simulink model "quad_tank_plant"  (R2026a)
settings: Solver=ode4  StopTime=inf
values from neighbouring files (symbols this model uses):
  a1 = (a11 + a12)/2    [areas.m]    (also in parametros.m = 0.0006136)
  A2 = 0.159    [parametros.m]
  a2 = mean([a21 a22],2)    [areas.m]    (also in parametros.m = 0.00054678)
  A3 = 0.159    [parametros.m]
  a3 = mean([a31 a32],2)    [areas.m]    (also in parametros.m = 0.00035752; prbs_calc_L3.m = 0.00035752; ti_calc.m = 0.00035752)
  A4 = 0.159    [parametros.m]
  a4 = mean([a41 a42],2)    [areas.m]    (also in parametros.m = 0.0004182; ti_calc.m = 0.0004182)
  g = 9.81    [areas.m]    (also in parametros.m; prbs_calc_L3.m; ti_calc.m)
  gamma1 = 0.455    [areas.m]    (also in parametros.m)
  gamma2 = 0.4195    [areas.m]    (also in parametros.m)
  h_max = 0.6    [areas.m]    (also in parametros.m)
  k1 = q_max    (= 0.0017)    [areas.m]    (also in parametros.m)
  k2 = q_max    (= 0.0017)    [areas.m]    (also in parametros.m)
  q_max = 0.0017    [areas.m]    (also in parametros.m)
undefined symbols (not defined in the file or in its folder): A1
libraries: opcualib x2
settings Model: Creator=agusc  LastModifiedBy=agusc

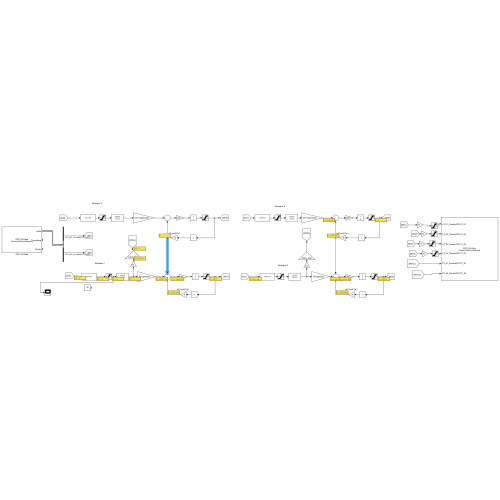
[thumbnail: Simulink's stored preview of the top-level diagram]
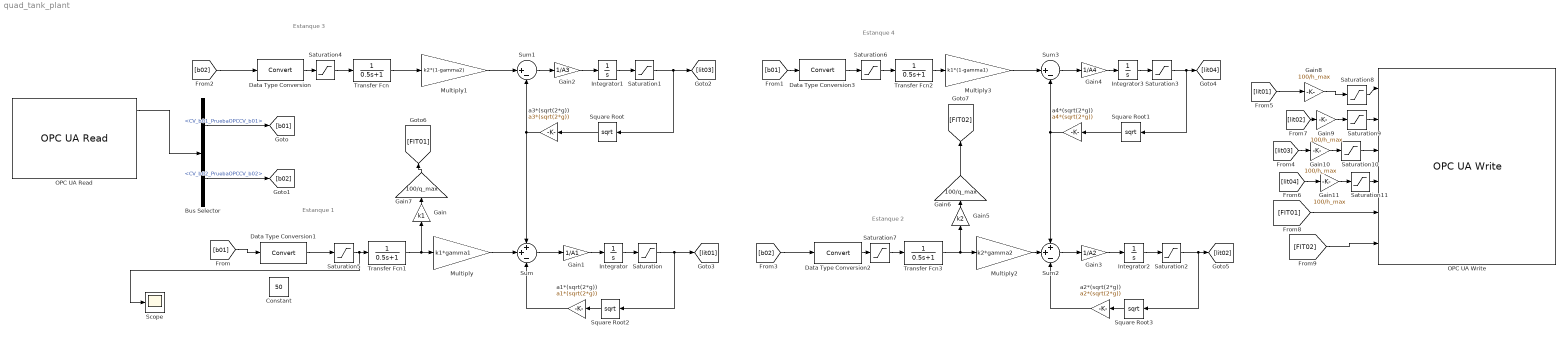
== system quad_tank_plant ==
  note: Estanque 2
  note: Estanque 4
  note: Estanque 3
  note: Estanque 1
  Bus Selector : BusSelector  OutputSignals=CV_b01_PruebaOPCCV_b01,CV_b02_PruebaOPCCV_b02
  Constant : Constant  Value=50
  Data Type Conversion{,1..3} (4 alike) : DataTypeConversion  SaturateOnIntegerOverflow=off  RndMeth=Floor
  Gain : Gain  Gain=k1
  Gain1 : Gain  Gain=1/A1
  Gain{8..11} (4 alike) : Gain  Gain=100/h_max
  Gain2 : Gain  Gain=1/A3
  Gain3 : Gain  Gain=1/A2
  Gain4 : Gain  Gain=1/A4
  Gain5 : Gain  Gain=k2
  Gain6 : Gain  Gain=100/q_max
  Gain7 : Gain  Gain=100/q_max
  Integrator{,1..3} (4 alike) : Integrator
  Multiply : Gain  Gain=k1*gamma1
  Multiply1 : Gain  Gain=k2*(1-gamma2)
  Multiply2 : Gain  Gain=k2*gamma2
  Multiply3 : Gain  Gain=k1*(1-gamma1)
  OPC UA Read : opcualib/OPC UA Read  SelectedServer=FactoryTalkLinxGateway  ServerList=FactoryTalkLinxGateway  NodeList={ '1', 'CV_b01', '2', '[Prueba OPC]CV_b01', 'off'; '2', 'CV_b02', '2', '[Prueba OPC]CV_b02', 'off' }  ShowQualityPort=on  ShowTimestampPort=on  ShowTimestampPortAs=Seconds since start  SampleTime=-1
  OPC UA Write : opcualib/OPC UA Write  SelectedServer=FactoryTalkLinxGateway  ServerList=FactoryTalkLinxGateway  SampleTime=-1  NodeList={ '1', 'LIT_01', '2', '[Prueba OPC]LIT_01', 'off'; '2', 'LIT_02', '2', '[Prueba OPC]LIT_02', 'off'; '3', 'LIT_03', '2', '[Prueba OPC]LIT_03', 'off'; '4', 'LIT_04', '2', '[Prueba OPC]LIT_04', 'off'; '5', 'FIT_01', '2', '[Prueba OPC]FIT_01', 'off'; '6', 'FIT_02', '2', '[Prueba OPC]FIT_02', 'off' }
  Saturation{,1..3} (4 alike) : Saturate  UpperLimit=h_max  LowerLimit=0
  Saturation{8..11} (4 alike) : Saturate  UpperLimit=100  LowerLimit=0
  Saturation{4..7} (4 alike) : Saturate  UpperLimit=50  LowerLimit=0
  Scope : Scope
      settings: ActiveDisplayYMinimum=40  ActiveDisplayYMaximum=60
  Square Root{,1..3} (4 alike) : Sqrt
  Sum : Sum  Inputs=++-
  Sum1 : Sum  Inputs=|+-
  Sum2 : Sum  Inputs=++-
  Sum3 : Sum  Inputs=|+-
  Transfer Fcn{,1..3} (4 alike) : TransferFcn  Denominator=[0.5 1]
  a1*(sqrt(2*g)) : Gain  Gain=a1*(sqrt(2*g))
  a2*(sqrt(2*g)) : Gain  Gain=a2*(sqrt(2*g))
  a3*(sqrt(2*g)) : Gain  Gain=a3*(sqrt(2*g))
  a4*(sqrt(2*g)) : Gain  Gain=a4*(sqrt(2*g))
  wires:
  Multiply/1 -> Sum/2
  Square Root/1 -> a3*(sqrt(2*g))/1
  a1*(sqrt(2*g))/1 -> Sum/3
  Square Root2/1 -> a1*(sqrt(2*g))/1
  Saturation1/1 -> [lit03], Square Root/1
  Multiply1/1 -> Sum1/1
  a3*(sqrt(2*g))/1 -> Sum/1, Sum1/2
  Saturation/1 -> [lit01], Square Root2/1
  Gain1/1 -> Integrator/1
  Multiply3/1 -> Sum3/1
  Saturation2/1 -> [lit02], Square Root3/1
  a4*(sqrt(2*g))/1 -> Sum2/1, Sum3/2
  Multiply2/1 -> Sum2/2
  a2*(sqrt(2*g))/1 -> Sum2/3
  Square Root1/1 -> a4*(sqrt(2*g))/1
  Sum2/1 -> Gain3/1
  Gain4/1 -> Integrator3/1
  Saturation3/1 -> [lit04], Square Root1/1
  Square Root3/1 -> a2*(sqrt(2*g))/1
  Sum1/1 -> Gain2/1
  Gain2/1 -> Integrator1/1
  Integrator1/1 -> Saturation1/1
  Sum/1 -> Gain1/1
  Integrator/1 -> Saturation/1
  Integrator2/1 -> Saturation2/1
  Gain3/1 -> Integrator2/1
  Sum3/1 -> Gain4/1
  Integrator3/1 -> Saturation3/1
  Saturation4/1 -> Transfer Fcn/1
  Transfer Fcn/1 -> Multiply1/1
  Saturation5/1 -> Scope/1, Transfer Fcn1/1
  Transfer Fcn1/1 -> Gain/1, Multiply/1
  Saturation6/1 -> Transfer Fcn2/1
  Transfer Fcn2/1 -> Multiply3/1
  Saturation7/1 -> Transfer Fcn3/1
  OPC UA Read/1 -> Bus Selector/1
  Bus Selector/1 -> [b01]  "<CV_b01_PruebaOPCCV_b01>"
  [b01] -> Data Type Conversion1/1
  [b01] -> Data Type Conversion3/1
  Bus Selector/2 -> [b02]  "<CV_b02_PruebaOPCCV_b02>"
  [lit03] -> Gain10/1
  [lit01] -> Gain8/1
  [lit04] -> Gain11/1
  [lit02] -> Gain9/1
  [FIT01] -> OPC UA Write/5
  Gain/1 -> Gain7/1
  Transfer Fcn3/1 -> Gain5/1, Multiply2/1
  Gain5/1 -> Gain6/1
  [FIT02] -> OPC UA Write/6
  Data Type Conversion/1 -> Saturation4/1
  Data Type Conversion2/1 -> Saturation7/1
  Data Type Conversion3/1 -> Saturation6/1
  Gain6/1 -> [FIT02]
  Gain7/1 -> [FIT01]
  Gain8/1 -> Saturation8/1
  Gain9/1 -> Saturation9/1
  Gain10/1 -> Saturation10/1
  Gain11/1 -> Saturation11/1
  Saturation8/1 -> OPC UA Write/1
  Saturation9/1 -> OPC UA Write/2
  Saturation10/1 -> OPC UA Write/3
  Saturation11/1 -> OPC UA Write/4
  Data Type Conversion1/1 -> Saturation5/1
  [b02] -> Data Type Conversion2/1
  [b02] -> Data Type Conversion/1
